simulink subsystem "tehrani_lung_compartment"  (R2019b)
settings: Solver=VariableStepAuto  StartTime=0.0  StopTime=10.0  RelTol=1e-3
settings Model: Creator=RH  LastModifiedBy=RH

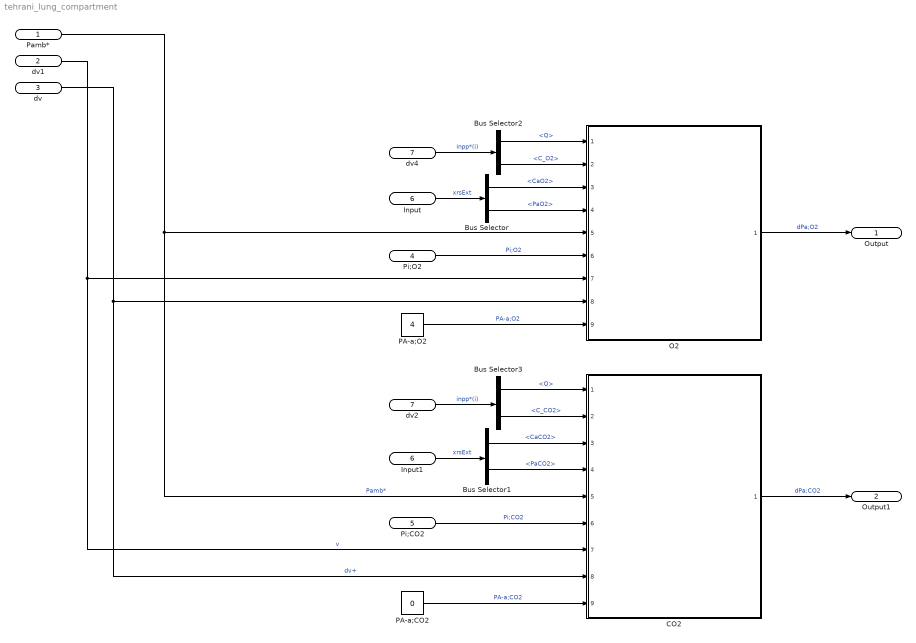
== system tehrani_lung_compartment ==
  Pamb* : Inport  Unit=mmHg
  dv1 : Inport  Port=2  Unit=L
  dv : Inport  Port=3  Unit=L/s
  Pi;O2 : Inport  Port=4  Unit=mmHg
  Pi;CO2 : Inport  Port=5  Unit=mmHg
  Input : Inport  Port=6  OutDataTypeStr=Bus: RespiratoryStateExtended
  dv4 : Inport  Port=7  OutDataTypeStr=Bus: BloodGasFlow
  Bus Selector : BusSelector  OutputSignals=CaO2,PaO2
  Bus Selector1 : BusSelector  OutputSignals=CaCO2,PaCO2
  Bus Selector2 : BusSelector  OutputSignals=Q,C_O2
  Bus Selector3 : BusSelector  OutputSignals=Q,C_CO2
  CO2 : Subsystem  ReferencedSubsystem=tehrani_alv_mass_balance_v5
  Input1 : InportShadow  Port=6  OutDataTypeStr=Bus: RespiratoryStateExtended
  O2 : Subsystem  ReferencedSubsystem=tehrani_alv_mass_balance_v5
  PA-a;CO2 : Constant  Value=0
  PA-a;O2 : Constant  Value=4
  dv2 : InportShadow  Port=7  OutDataTypeStr=Bus: BloodGasFlow
  Output : Outport  Unit=mmHg/s
  Output1 : Outport  Port=2  Unit=mmHg/s
  wires:
  dv1/1 -> O2/7, CO2/7  "v"
  Pamb*/1 -> O2/5, CO2/5  "Pamb*"
  dv/1 -> O2/8, CO2/8  "dv+"
  Pi;O2/1 -> O2/6  "Pi;O2"
  PA-a;O2/1 -> O2/9  "PA-a;O2"
  Input/1 -> Bus Selector/1  "xrsExt"
  Bus Selector/2 -> O2/4  "<PaO2>"
  Bus Selector/1 -> O2/3  "<CaO2>"
  O2/1 -> Output/1  "dPa;O2"
  CO2/1 -> Output1/1  "dPa;CO2"
  Input1/1 -> Bus Selector1/1  "xrsExt"
  Bus Selector3/2 -> CO2/2  "<C_CO2>"
  Bus Selector3/1 -> CO2/1  "<Q>"
  Pi;CO2/1 -> CO2/6  "Pi;CO2"
  PA-a;CO2/1 -> CO2/9  "PA-a;CO2"
  dv4/1 -> Bus Selector2/1  "inpp*(i)"
  Bus Selector2/1 -> O2/1  "<Q>"
  Bus Selector2/2 -> O2/2  "<C_O2>"
  Bus Selector1/1 -> CO2/3  "<CaCO2>"
  Bus Selector1/2 -> CO2/4  "<PaCO2>"
  dv2/1 -> Bus Selector3/1  "inpp*(i)"
